simulink model "testMatlabFunction"  (Simulink 8.3)
settings: Solver=ode45  StartTime=0.0  StopTime=100  RelTol=1e-3
settings Model: Creator=shawn  LastModifiedBy=scorpii  CovSFcnEnable=on
settings DataIOCC: SignalLoggingSaveFormat=Dataset
settings DebuggingCC: UnderspecifiedInitializationDetection=Simplified  MergeDetectMultiDrivingBlocksExec=error  SolverPrmCheckMsg=none  FrameProcessingCompatibilityMsg=error  StateNameClashWarn=none
settings GRTTargetCC: CombineOutputUpdateFcns=on  GRTInterface=off

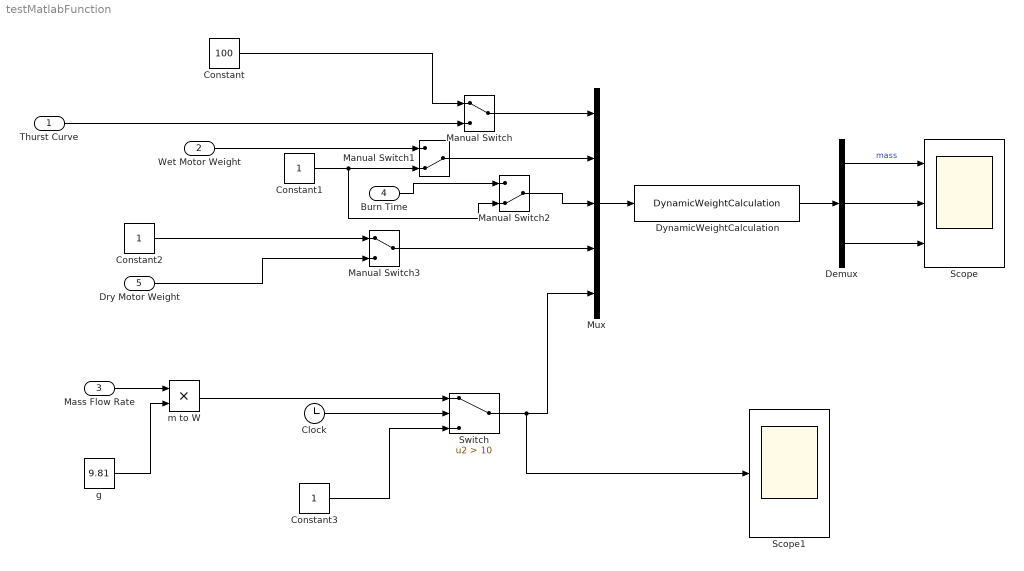
== system testMatlabFunction ==
  Thurst Curve : Inport
  Wet Motor Weight : Inport  Port=2
  Mass Flow Rate : Inport  Port=3
  Burn Time : Inport  Port=4
  Dry Motor Weight : Inport  Port=5
  Clock : Clock
  Constant : Constant  Value=100
  Constant1 : Constant
  Constant2 : Constant
  Constant3 : Constant
  Demux : Demux  Outputs=[1 1 1]
  DynamicWeightCalculation : MATLABFcn  MATLABFcn=DynamicWeightCalculation
      mask Display: disp('DynamicWeightCalculation')
  Manual Switch : ManualSwitch
  Manual Switch1 : ManualSwitch  CurrentSetting=0
  Manual Switch2 : ManualSwitch  CurrentSetting=0
  Manual Switch3 : ManualSwitch
  Mux : Mux  Inputs=5
  Scope : Scope  NumInputPorts=3
      settings: YMin=-5~-5~-5  YMax=5~5~5
  Scope1 : Scope
  Switch : Switch  Criteria=u2 > Threshold  Threshold=10
  g : Constant  Value=9.81
  m to W : Product
  wires:
  g/1 -> m to W/2
  Mass Flow Rate/1 -> m to W/1
  Mux/1 -> DynamicWeightCalculation/1
  DynamicWeightCalculation/1 -> Demux/1
  Demux/1 -> Scope/1  "mass"
  Demux/2 -> Scope/2
  Demux/3 -> Scope/3
  Constant/1 -> Manual Switch/1
  Manual Switch/1 -> Mux/1
  Thurst Curve/1 -> Manual Switch/2
  Manual Switch1/1 -> Mux/2
  Manual Switch2/1 -> Mux/3
  Constant1/1 -> Manual Switch2/2, Manual Switch1/2
  Manual Switch3/1 -> Mux/4
  Switch/1 -> Scope1/1, Mux/5
  Wet Motor Weight/1 -> Manual Switch1/1
  Dry Motor Weight/1 -> Manual Switch3/2
  m to W/1 -> Switch/1
  Burn Time/1 -> Manual Switch2/1
  Constant2/1 -> Manual Switch3/1
  Constant3/1 -> Switch/3
  Clock/1 -> Switch/2
